simulink model "Pedal_Interpretation_exe"  (Simulink 7.0)
settings: Solver=ode4  StartTime=0.0  StopTime=88  FixedStep=0.01  RelTol=1e-3
InitFcn:
  | PedalInterp_para
values from neighbouring files (symbols this model uses):
  ped_min = 5    [PedalInterp_para.m]
  T_max_Brake = 4000    [PedalInterp_para.m]
  TI = 0    [PAS_callback.m]
undefined symbols (not defined in the file or in its folder): fzgbib, m_ab_100pro, m_ab_70pro, PedalInterpretation, v_bereich
libraries: simulink x320
(part 8 of 23)

== system Pedal_Interpretation_exe/Validation Functions/SR-PI-02.2 Acceleration pedal interpretation/v = const & phi_Acc increases & T_des_Drive < 0/PS ==
  A TI1 : Inport  OutDataType=sfix(16)  OutScaling=2^0
  A TI2 : Inport  Port=2  OutDataType=sfix(16)  OutScaling=2^0
  A TI3 : Inport  Port=3  OutDataType=sfix(16)  OutScaling=2^0
  AND : Logic  Inputs=4  AllPortsSameDT=off  OutDataTypeMode=boolean
  Bus Creator : BusCreator  Inputs=3
  Data Type Conversion : DataTypeConversion  OutDataType=sfix(16)  OutScaling=2^0
  Data Type Conversion1 : DataTypeConversion  OutDataType=sfix(16)  OutScaling=2^0
  Data Type Conversion2 : DataTypeConversion  OutDataType=sfix(16)  OutScaling=2^0
  Max Delay A : Subsystem  TreatAsAtomicUnit=on  mask{Delay=2}
      mask prompts: Delay "Delay (in simulation steps) for the input signal:"
      mask init:
      | %set_param([gcb '/Discrete Transfer Fcn'],'Denominator',['[' num2str([1 zeros(1,str2double(get_param(gcb,'Delay')))]) ']']);
      mask CallbackString:
      | Delay = str2double(get_param(gcb,'Delay'));
      | if Delay < 0
      |     set_param(gcb,'Delay','0');
      |     error('Only non-negative delays are possible (causality).');
      |     set_param([gcb '/Delay'],'Value','0');
      | elseif Delay == 0
      |     set_param([gcb '/Delay'],'Value','0');
      | else
      |     set_param([gcb '/Integer Delay'],'NumDelays',num2str(Delay));
      |     set_param([gcb '/Delay'],'Value',num2str(Delay));
      | end
      mask Display: text(0.5,0.5,['z^{ ' num2str((-1)*str2double(get_param(gcb,'Delay'))) '}'],'texmode','on');
  Max Delay R : Subsystem  TreatAsAtomicUnit=on  mask{Delay=2}
      mask prompts: Delay "Delay (in simulation steps) for the input signal:"
      mask init:
      | %set_param([gcb '/Discrete Transfer Fcn'],'Denominator',['[' num2str([1 zeros(1,str2double(get_param(gcb,'Delay')))]) ']']);
      mask CallbackString:
      | Delay = str2double(get_param(gcb,'Delay'));
      | if Delay < 0
      |     set_param(gcb,'Delay','0');
      |     error('Only non-negative delays are possible (causality).');
      |     set_param([gcb '/Delay'],'Value','0');
      | elseif Delay == 0
      |     set_param([gcb '/Delay'],'Value','0');
      | else
      |     set_param([gcb '/Integer Delay'],'NumDelays',num2str(Delay));
      |     set_param([gcb '/Delay'],'Value',num2str(Delay));
      | end
      mask Display: text(0.5,0.5,['z^{ ' num2str((-1)*str2double(get_param(gcb,'Delay'))) '}'],'texmode','on');
  Max Delay T : Subsystem  TreatAsAtomicUnit=on  mask{Delay=2}
      mask prompts: Delay "Delay (in simulation steps) for the input signal:"
      mask init:
      | %set_param([gcb '/Discrete Transfer Fcn'],'Denominator',['[' num2str([1 zeros(1,str2double(get_param(gcb,'Delay')))]) ']']);
      mask CallbackString:
      | Delay = str2double(get_param(gcb,'Delay'));
      | if Delay < 0
      |     set_param(gcb,'Delay','0');
      |     error('Only non-negative delays are possible (causality).');
      |     set_param([gcb '/Delay'],'Value','0');
      | elseif Delay == 0
      |     set_param([gcb '/Delay'],'Value','0');
      | else
      |     set_param([gcb '/Integer Delay'],'NumDelays',num2str(Delay));
      |     set_param([gcb '/Delay'],'Value',num2str(Delay));
      | end
      mask Display: text(0.5,0.5,['z^{ ' num2str((-1)*str2double(get_param(gcb,'Delay'))) '}'],'texmode','on');
  OR - AND : Subsystem
  TDD : Subsystem
  TI : Subsystem
  TID : Subsystem
  Precond : Outport  OutDataType=sfix(16)  OutScaling=2^0
  wires:
  TDD/2(T) -> AND/4
  TID/2(T) -> Max Delay T/1(In1)
  TID/1(A) -> Max Delay A/1(In1)
  Bus Creator/1 -> Precond/1
  Data Type Conversion/1 -> Bus Creator/1  "A"
  Data Type Conversion1/1 -> Bus Creator/2  "T"
  TDD/1(A) -> AND/3
  Max Delay T/1(Out1) -> Data Type Conversion1/1
  Max Delay R/1(Out1) -> AND/1
  Max Delay A/1(Out1) -> Data Type Conversion/1
  AND/1 -> Data Type Conversion2/1
  OR - AND/2(AND) -> TID/2(R AND), Max Delay R/1(In1)
  OR - AND/1(OR) -> TID/1(R OR)
  TI/1(A) -> AND/2
  Data Type Conversion2/1 -> Bus Creator/3  "R"
  A TI1/1 -> TI/1(A1)
  A TI2/1 -> TI/2(A2)
  A TI3/1 -> TI/3(A3)

== system Pedal_Interpretation_exe/Validation Functions/SR-PI-02.2 Acceleration pedal interpretation/v = const & phi_Acc increases & T_des_Drive < 0/Range - Gap Relative tolerance Precond ==
  Signal : Inport  OutDataType=sfix(16)  OutScaling=2^0
  Reference : Inport  Port=2  OutDataType=sfix(16)  OutScaling=2^0
  Abs : Abs
  Abs1 : Abs
  Add : Sum  Inputs=+-  OutDataType=sfix(16)  OutScaling=2^-10
  Divide1 : Product  Inputs=**/  OutDataType=sfix(16)  OutScaling=2^-10
  Max : Constant  Value=100  OutDataType=sfix(16)  OutScaling=2^0
  Relational Operator : RelationalOperator  Operator=<=  LogicOutDataTypeMode=boolean
  Relative Tolerance : Constant  OutDataType=sfix(16)  OutScaling=2^0
  Activate : Outport  OutDataType=sfix(16)  OutScaling=2^0
  wires:
  Abs/1 -> Relational Operator/1
  Add/1 -> Abs/1
  Signal/1 -> Add/1
  Reference/1 -> Add/2, Abs1/1
  Divide1/1 -> Relational Operator/2
  Max/1 -> Divide1/3
  Relative Tolerance/1 -> Divide1/2
  Relational Operator/1 -> Activate/1
  Abs1/1 -> Divide1/1

== system Pedal_Interpretation_exe/Validation Functions/SR-PI-02.2 Acceleration pedal interpretation/v = const & phi_Acc increases & T_des_Drive < 0/Range - Gap Relative tolerance Precond1 ==
  Signal : Inport  OutDataType=sfix(16)  OutScaling=2^0
  Reference : Inport  Port=2  OutDataType=sfix(16)  OutScaling=2^0
  Abs : Abs
  Abs1 : Abs
  Add : Sum  Inputs=+-  OutDataType=sfix(16)  OutScaling=2^-10
  Divide1 : Product  Inputs=**/  OutDataType=sfix(16)  OutScaling=2^-10
  Max : Constant  Value=100  OutDataType=sfix(16)  OutScaling=2^0
  Relational Operator : RelationalOperator  Operator=<=  LogicOutDataTypeMode=boolean
  Relative Tolerance : Constant  OutDataType=sfix(16)  OutScaling=2^0
  Activate : Outport  OutDataType=sfix(16)  OutScaling=2^0
  wires:
  Abs/1 -> Relational Operator/1
  Add/1 -> Abs/1
  Signal/1 -> Add/1
  Reference/1 -> Add/2, Abs1/1
  Divide1/1 -> Relational Operator/2
  Max/1 -> Divide1/3
  Relative Tolerance/1 -> Divide1/2
  Relational Operator/1 -> Activate/1
  Abs1/1 -> Divide1/1

== system Pedal_Interpretation_exe/Validation Functions/SR-PI-02.2 Acceleration pedal interpretation/v = const & phi_Acc increases & T_des_Drive >= 0/Bound Precond ==
  Signal : Inport  OutDataType=sfix(16)  OutScaling=2^0
  Reference : Inport  Port=2  OutDataType=sfix(16)  OutScaling=2^0
  RelOp : RelationalOperator  LogicOutDataTypeMode=Specify via dialog
  Activate : Outport  OutDataType=sfix(16)  OutScaling=2^0
  wires:
  Reference/1 -> RelOp/2
  RelOp/1 -> Activate/1
  Signal/1 -> RelOp/1

== system Pedal_Interpretation_exe/Validation Functions/SR-PI-02.2 Acceleration pedal interpretation/v = const & phi_Acc increases & T_des_Drive >= 0/Detect constant ==
  Signal : Inport  OutDataType=sfix(16)  OutScaling=2^0
  Clock : Clock
      settings: Decimation=10
  Constant1 : Constant  Value=0  OutDataTypeMode=boolean  OutDataType=sfix(16)  OutScaling=2^0
  Memory : Memory
  Relative tolerance : Subsystem
  Switch : Switch  Criteria=u2 > Threshold
  Constant : Outport  OutDataType=sfix(16)  OutScaling=2^0
  wires:
  Signal/1 -> Memory/1, Relative tolerance/1(sig)
  Memory/1 -> Relative tolerance/2(ref)
  Constant1/1 -> Switch/3
  Clock/1 -> Switch/2
  Relative tolerance/1(sig == ref) -> Switch/1
  Switch/1 -> Constant/1

== system Pedal_Interpretation_exe/Validation Functions/SR-PI-02.2 Acceleration pedal interpretation/v = const & phi_Acc increases & T_des_Drive >= 0/Detect increase ==
  Signal : Inport  OutDataType=sfix(16)  OutScaling=2^0
  Clock : Clock
      settings: Decimation=10
  Memory : Memory
  Relational Operator : RelationalOperator  Operator=>  LogicOutDataTypeMode=Specify via dialog
  Switch : Switch  Criteria=u2 > Threshold
  Increase : Outport  OutDataType=sfix(16)  OutScaling=2^0
  wires:
  Signal/1 -> Relational Operator/1, Memory/1, Switch/3
  Relational Operator/1 -> Increase/1
  Clock/1 -> Switch/2
  Memory/1 -> Switch/1
  Switch/1 -> Relational Operator/2

== system Pedal_Interpretation_exe/Validation Functions/SR-PI-02.2 Acceleration pedal interpretation/v = const & phi_Acc increases & T_des_Drive >= 0/PS ==
  A TI1 : Inport  OutDataType=sfix(16)  OutScaling=2^0
  A TI2 : Inport  Port=2  OutDataType=sfix(16)  OutScaling=2^0
  A TI3 : Inport  Port=3  OutDataType=sfix(16)  OutScaling=2^0
  AND : Logic  Inputs=4  AllPortsSameDT=off  OutDataTypeMode=boolean
  Bus Creator : BusCreator  Inputs=3
  Data Type Conversion : DataTypeConversion  OutDataType=sfix(16)  OutScaling=2^0
  Data Type Conversion1 : DataTypeConversion  OutDataType=sfix(16)  OutScaling=2^0
  Data Type Conversion2 : DataTypeConversion  OutDataType=sfix(16)  OutScaling=2^0
  Max Delay A : Subsystem  TreatAsAtomicUnit=on  mask{Delay=2}
      mask prompts: Delay "Delay (in simulation steps) for the input signal:"
      mask init:
      | %set_param([gcb '/Discrete Transfer Fcn'],'Denominator',['[' num2str([1 zeros(1,str2double(get_param(gcb,'Delay')))]) ']']);
      mask CallbackString:
      | Delay = str2double(get_param(gcb,'Delay'));
      | if Delay < 0
      |     set_param(gcb,'Delay','0');
      |     error('Only non-negative delays are possible (causality).');
      |     set_param([gcb '/Delay'],'Value','0');
      | elseif Delay == 0
      |     set_param([gcb '/Delay'],'Value','0');
      | else
      |     set_param([gcb '/Integer Delay'],'NumDelays',num2str(Delay));
      |     set_param([gcb '/Delay'],'Value',num2str(Delay));
      | end
      mask Display: text(0.5,0.5,['z^{ ' num2str((-1)*str2double(get_param(gcb,'Delay'))) '}'],'texmode','on');
  Max Delay R : Subsystem  TreatAsAtomicUnit=on  mask{Delay=2}
      mask prompts: Delay "Delay (in simulation steps) for the input signal:"
      mask init:
      | %set_param([gcb '/Discrete Transfer Fcn'],'Denominator',['[' num2str([1 zeros(1,str2double(get_param(gcb,'Delay')))]) ']']);
      mask CallbackString:
      | Delay = str2double(get_param(gcb,'Delay'));
      | if Delay < 0
      |     set_param(gcb,'Delay','0');
      |     error('Only non-negative delays are possible (causality).');
      |     set_param([gcb '/Delay'],'Value','0');
      | elseif Delay == 0
      |     set_param([gcb '/Delay'],'Value','0');
      | else
      |     set_param([gcb '/Integer Delay'],'NumDelays',num2str(Delay));
      |     set_param([gcb '/Delay'],'Value',num2str(Delay));
      | end
      mask Display: text(0.5,0.5,['z^{ ' num2str((-1)*str2double(get_param(gcb,'Delay'))) '}'],'texmode','on');
  Max Delay T : Subsystem  TreatAsAtomicUnit=on  mask{Delay=2}
      mask prompts: Delay "Delay (in simulation steps) for the input signal:"
      mask init:
      | %set_param([gcb '/Discrete Transfer Fcn'],'Denominator',['[' num2str([1 zeros(1,str2double(get_param(gcb,'Delay')))]) ']']);
      mask CallbackString:
      | Delay = str2double(get_param(gcb,'Delay'));
      | if Delay < 0
      |     set_param(gcb,'Delay','0');
      |     error('Only non-negative delays are possible (causality).');
      |     set_param([gcb '/Delay'],'Value','0');
      | elseif Delay == 0
      |     set_param([gcb '/Delay'],'Value','0');
      | else
      |     set_param([gcb '/Integer Delay'],'NumDelays',num2str(Delay));
      |     set_param([gcb '/Delay'],'Value',num2str(Delay));
      | end
      mask Display: text(0.5,0.5,['z^{ ' num2str((-1)*str2double(get_param(gcb,'Delay'))) '}'],'texmode','on');
  OR - AND : Subsystem
  TDD : Subsystem
  TI : Subsystem
  TID : Subsystem
  Precond : Outport  OutDataType=sfix(16)  OutScaling=2^0
  wires:
  TDD/2(T) -> AND/4
  TID/2(T) -> Max Delay T/1(In1)
  TID/1(A) -> Max Delay A/1(In1)
  Bus Creator/1 -> Precond/1
  Data Type Conversion/1 -> Bus Creator/1  "A"
  Data Type Conversion1/1 -> Bus Creator/2  "T"
  TDD/1(A) -> AND/3
  Max Delay T/1(Out1) -> Data Type Conversion1/1
  Max Delay R/1(Out1) -> AND/1
  Max Delay A/1(Out1) -> Data Type Conversion/1
  AND/1 -> Data Type Conversion2/1
  OR - AND/2(AND) -> TID/2(R AND), Max Delay R/1(In1)
  OR - AND/1(OR) -> TID/1(R OR)
  TI/1(A) -> AND/2
  Data Type Conversion2/1 -> Bus Creator/3  "R"
  A TI1/1 -> TI/1(A1)
  A TI2/1 -> TI/2(A2)
  A TI3/1 -> TI/3(A3)

== system Pedal_Interpretation_exe/Validation Functions/SR-PI-02.2 Acceleration pedal interpretation/v = const & phi_Acc increases & T_des_Drive >= 0/Range - Gap Relative tolerance Precond ==
  Signal : Inport  OutDataType=sfix(16)  OutScaling=2^0
  Reference : Inport  Port=2  OutDataType=sfix(16)  OutScaling=2^0
  Abs : Abs
  Abs1 : Abs
  Add : Sum  Inputs=+-  OutDataType=sfix(16)  OutScaling=2^-10
  Divide1 : Product  Inputs=**/  OutDataType=sfix(16)  OutScaling=2^-10
  Max : Constant  Value=100  OutDataType=sfix(16)  OutScaling=2^0
  Relational Operator : RelationalOperator  Operator=<=  LogicOutDataTypeMode=boolean
  Relative Tolerance : Constant  OutDataType=sfix(16)  OutScaling=2^0
  Activate : Outport  OutDataType=sfix(16)  OutScaling=2^0
  wires:
  Abs/1 -> Relational Operator/1
  Add/1 -> Abs/1
  Signal/1 -> Add/1
  Reference/1 -> Add/2, Abs1/1
  Divide1/1 -> Relational Operator/2
  Max/1 -> Divide1/3
  Relative Tolerance/1 -> Divide1/2
  Relational Operator/1 -> Activate/1
  Abs1/1 -> Divide1/1

== system Pedal_Interpretation_exe/Validation Functions/SR-PI-02.2 Acceleration pedal interpretation/v = const & phi_Acc increases & T_des_Drive >= 0/Range - Gap Relative tolerance Precond1 ==
  Signal : Inport  OutDataType=sfix(16)  OutScaling=2^0
  Reference : Inport  Port=2  OutDataType=sfix(16)  OutScaling=2^0
  Abs : Abs
  Abs1 : Abs
  Add : Sum  Inputs=+-  OutDataType=sfix(16)  OutScaling=2^-10
  Divide1 : Product  Inputs=**/  OutDataType=sfix(16)  OutScaling=2^-10
  Max : Constant  Value=100  OutDataType=sfix(16)  OutScaling=2^0
  Relational Operator : RelationalOperator  Operator=<=  LogicOutDataTypeMode=boolean
  Relative Tolerance : Constant  OutDataType=sfix(16)  OutScaling=2^0
  Activate : Outport  OutDataType=sfix(16)  OutScaling=2^0
  wires:
  Abs/1 -> Relational Operator/1
  Add/1 -> Abs/1
  Signal/1 -> Add/1
  Reference/1 -> Add/2, Abs1/1
  Divide1/1 -> Relational Operator/2
  Max/1 -> Divide1/3
  Relative Tolerance/1 -> Divide1/2
  Relational Operator/1 -> Activate/1
  Abs1/1 -> Divide1/1

== system Pedal_Interpretation_exe/Validation Functions/SR-PI-02.2 Acceleration pedal interpretation/v increases & phi_Acc = const & T_des_Drive >= 0/Bound Precond ==
  Signal : Inport  OutDataType=sfix(16)  OutScaling=2^0
  Reference : Inport  Port=2  OutDataType=sfix(16)  OutScaling=2^0
  RelOp : RelationalOperator  LogicOutDataTypeMode=Specify via dialog
  Activate : Outport  OutDataType=sfix(16)  OutScaling=2^0
  wires:
  Reference/1 -> RelOp/2
  RelOp/1 -> Activate/1
  Signal/1 -> RelOp/1

== system Pedal_Interpretation_exe/Validation Functions/SR-PI-02.2 Acceleration pedal interpretation/v increases & phi_Acc = const & T_des_Drive >= 0/Detect constant ==
  Signal : Inport  OutDataType=sfix(16)  OutScaling=2^0
  Clock : Clock
      settings: Decimation=10
  Constant1 : Constant  Value=0  OutDataTypeMode=boolean  OutDataType=sfix(16)  OutScaling=2^0
  Memory : Memory
  Relative tolerance : Subsystem
  Switch : Switch  Criteria=u2 > Threshold
  Constant : Outport  OutDataType=sfix(16)  OutScaling=2^0
  wires:
  Signal/1 -> Memory/1, Relative tolerance/1(sig)
  Memory/1 -> Relative tolerance/2(ref)
  Constant1/1 -> Switch/3
  Clock/1 -> Switch/2
  Relative tolerance/1(sig == ref) -> Switch/1
  Switch/1 -> Constant/1

== system Pedal_Interpretation_exe/Validation Functions/SR-PI-02.2 Acceleration pedal interpretation/v increases & phi_Acc = const & T_des_Drive >= 0/Detect increase ==
  Signal : Inport  OutDataType=sfix(16)  OutScaling=2^0
  Clock : Clock
      settings: Decimation=10
  Memory : Memory
  Relational Operator : RelationalOperator  Operator=>  LogicOutDataTypeMode=Specify via dialog
  Switch : Switch  Criteria=u2 > Threshold
  Increase : Outport  OutDataType=sfix(16)  OutScaling=2^0
  wires:
  Signal/1 -> Relational Operator/1, Memory/1, Switch/3
  Relational Operator/1 -> Increase/1
  Clock/1 -> Switch/2
  Memory/1 -> Switch/1
  Switch/1 -> Relational Operator/2

== system Pedal_Interpretation_exe/Validation Functions/SR-PI-02.2 Acceleration pedal interpretation/v increases & phi_Acc = const & T_des_Drive >= 0/PS ==
  A TI1 : Inport  OutDataType=sfix(16)  OutScaling=2^0
  A TI2 : Inport  Port=2  OutDataType=sfix(16)  OutScaling=2^0
  A TI3 : Inport  Port=3  OutDataType=sfix(16)  OutScaling=2^0
  AND : Logic  Inputs=4  AllPortsSameDT=off  OutDataTypeMode=boolean
  Bus Creator : BusCreator  Inputs=3
  Data Type Conversion : DataTypeConversion  OutDataType=sfix(16)  OutScaling=2^0
  Data Type Conversion1 : DataTypeConversion  OutDataType=sfix(16)  OutScaling=2^0
  Data Type Conversion2 : DataTypeConversion  OutDataType=sfix(16)  OutScaling=2^0
  Max Delay A : Subsystem  TreatAsAtomicUnit=on  mask{Delay=2}
      mask prompts: Delay "Delay (in simulation steps) for the input signal:"
      mask init:
      | %set_param([gcb '/Discrete Transfer Fcn'],'Denominator',['[' num2str([1 zeros(1,str2double(get_param(gcb,'Delay')))]) ']']);
      mask CallbackString:
      | Delay = str2double(get_param(gcb,'Delay'));
      | if Delay < 0
      |     set_param(gcb,'Delay','0');
      |     error('Only non-negative delays are possible (causality).');
      |     set_param([gcb '/Delay'],'Value','0');
      | elseif Delay == 0
      |     set_param([gcb '/Delay'],'Value','0');
      | else
      |     set_param([gcb '/Integer Delay'],'NumDelays',num2str(Delay));
      |     set_param([gcb '/Delay'],'Value',num2str(Delay));
      | end
      mask Display: text(0.5,0.5,['z^{ ' num2str((-1)*str2double(get_param(gcb,'Delay'))) '}'],'texmode','on');
  Max Delay R : Subsystem  TreatAsAtomicUnit=on  mask{Delay=2}
      mask prompts: Delay "Delay (in simulation steps) for the input signal:"
      mask init:
      | %set_param([gcb '/Discrete Transfer Fcn'],'Denominator',['[' num2str([1 zeros(1,str2double(get_param(gcb,'Delay')))]) ']']);
      mask CallbackString:
      | Delay = str2double(get_param(gcb,'Delay'));
      | if Delay < 0
      |     set_param(gcb,'Delay','0');
      |     error('Only non-negative delays are possible (causality).');
      |     set_param([gcb '/Delay'],'Value','0');
      | elseif Delay == 0
      |     set_param([gcb '/Delay'],'Value','0');
      | else
      |     set_param([gcb '/Integer Delay'],'NumDelays',num2str(Delay));
      |     set_param([gcb '/Delay'],'Value',num2str(Delay));
      | end
      mask Display: text(0.5,0.5,['z^{ ' num2str((-1)*str2double(get_param(gcb,'Delay'))) '}'],'texmode','on');
  Max Delay T : Subsystem  TreatAsAtomicUnit=on  mask{Delay=2}
      mask prompts: Delay "Delay (in simulation steps) for the input signal:"
      mask init:
      | %set_param([gcb '/Discrete Transfer Fcn'],'Denominator',['[' num2str([1 zeros(1,str2double(get_param(gcb,'Delay')))]) ']']);
      mask CallbackString:
      | Delay = str2double(get_param(gcb,'Delay'));
      | if Delay < 0
      |     set_param(gcb,'Delay','0');
      |     error('Only non-negative delays are possible (causality).');
      |     set_param([gcb '/Delay'],'Value','0');
      | elseif Delay == 0
      |     set_param([gcb '/Delay'],'Value','0');
      | else
      |     set_param([gcb '/Integer Delay'],'NumDelays',num2str(Delay));
      |     set_param([gcb '/Delay'],'Value',num2str(Delay));
      | end
      mask Display: text(0.5,0.5,['z^{ ' num2str((-1)*str2double(get_param(gcb,'Delay'))) '}'],'texmode','on');
  OR - AND : Subsystem
  TDD : Subsystem
  TI : Subsystem
  TID : Subsystem
  Precond : Outport  OutDataType=sfix(16)  OutScaling=2^0
  wires:
  TDD/2(T) -> AND/4
  TID/2(T) -> Max Delay T/1(In1)
  TID/1(A) -> Max Delay A/1(In1)
  Bus Creator/1 -> Precond/1
  Data Type Conversion/1 -> Bus Creator/1  "A"
  Data Type Conversion1/1 -> Bus Creator/2  "T"
  TDD/1(A) -> AND/3
  Max Delay T/1(Out1) -> Data Type Conversion1/1
  Max Delay R/1(Out1) -> AND/1
  Max Delay A/1(Out1) -> Data Type Conversion/1
  AND/1 -> Data Type Conversion2/1
  OR - AND/2(AND) -> TID/2(R AND), Max Delay R/1(In1)
  OR - AND/1(OR) -> TID/1(R OR)
  TI/1(A) -> AND/2
  Data Type Conversion2/1 -> Bus Creator/3  "R"
  A TI1/1 -> TI/1(A1)
  A TI2/1 -> TI/2(A2)
  A TI3/1 -> TI/3(A3)

== system Pedal_Interpretation_exe/Validation Functions/SR-PI-02.2 Acceleration pedal interpretation/v increases & phi_Acc = const & T_des_Drive >= 0/Range - Gap Relative tolerance Precond ==
  Signal : Inport  OutDataType=sfix(16)  OutScaling=2^0
  Reference : Inport  Port=2  OutDataType=sfix(16)  OutScaling=2^0
  Abs : Abs
  Abs1 : Abs
  Add : Sum  Inputs=+-  OutDataType=sfix(16)  OutScaling=2^-10
  Divide1 : Product  Inputs=**/  OutDataType=sfix(16)  OutScaling=2^-10
  Max : Constant  Value=100  OutDataType=sfix(16)  OutScaling=2^0
  Relational Operator : RelationalOperator  Operator=<=  LogicOutDataTypeMode=boolean
  Relative Tolerance : Constant  OutDataType=sfix(16)  OutScaling=2^0
  Activate : Outport  OutDataType=sfix(16)  OutScaling=2^0
  wires:
  Abs/1 -> Relational Operator/1
  Add/1 -> Abs/1
  Signal/1 -> Add/1
  Reference/1 -> Add/2, Abs1/1
  Divide1/1 -> Relational Operator/2
  Max/1 -> Divide1/3
  Relative Tolerance/1 -> Divide1/2
  Relational Operator/1 -> Activate/1
  Abs1/1 -> Divide1/1

== system Pedal_Interpretation_exe/Validation Functions/SR-PI-02.2 Acceleration pedal interpretation/v increases & phi_Acc = const & T_des_Drive >= 0/Range - Gap Relative tolerance Precond1 ==
  Signal : Inport  OutDataType=sfix(16)  OutScaling=2^0
  Reference : Inport  Port=2  OutDataType=sfix(16)  OutScaling=2^0
  Abs : Abs
  Abs1 : Abs
  Add : Sum  Inputs=+-  OutDataType=sfix(16)  OutScaling=2^-10
  Divide1 : Product  Inputs=**/  OutDataType=sfix(16)  OutScaling=2^-10
  Max : Constant  Value=100  OutDataType=sfix(16)  OutScaling=2^0
  Relational Operator : RelationalOperator  Operator=<=  LogicOutDataTypeMode=boolean
  Relative Tolerance : Constant  OutDataType=sfix(16)  OutScaling=2^0
  Activate : Outport  OutDataType=sfix(16)  OutScaling=2^0
  wires:
  Abs/1 -> Relational Operator/1
  Add/1 -> Abs/1
  Signal/1 -> Add/1
  Reference/1 -> Add/2, Abs1/1
  Divide1/1 -> Relational Operator/2
  Max/1 -> Divide1/3
  Relative Tolerance/1 -> Divide1/2
  Relational Operator/1 -> Activate/1
  Abs1/1 -> Divide1/1

== system Pedal_Interpretation_exe/TestData 1/SR-PI-01.1 Brake Pedal recognition/phi_Brake < ped_min/Generate decrease 2/Generate  limited decrease for partition1 variant1 1 ==
  Repeating Sequence : Subsystem  mask(Repeating table){rep_seq_t=[0 T], rep_seq_y=[X0 XF]}
      mask prompts: rep_seq_t "Time values:"; rep_seq_y "Output values:"
      mask help: Output a repeating sequence of numbers specified in a table of time-value pairs. Values of time should be monotonically increasing.
      mask init:
      | if (length(rep_seq_t) ~= length(rep_seq_y)),
      |   error('Length of time vector and output vector must be the same.')
      | end
      | dbl_rep_seq_t = double(rep_seq_t);
      | dbl_rep_seq_y = double(rep_seq_y);
      | period = max(dbl_rep_seq_t) - min(dbl_rep_seq_t);
      | s = round(length(dbl_rep_seq_t)/50);
      | if s > 0
      |   pts = [1:s:length(dbl_rep_seq_t)];
      |   L   = length(pts);
      | else
      |   L   = length(dbl_rep_seq_t);
      |   pts = [1:L];
      | end
      | 
      | disp_seq_t = reshape(dbl_rep_seq_t(pts),L,1);
      | disp_seq_y = reshape(dbl_rep_seq_y(pts),L,1);
      | disp_period = max(disp_seq_t) - min(disp_seq_t);
      | 
      | disp_seq_t  = repmat(disp_seq_t,1,3) + (ones(L,1)*(disp_period*[0,1,2]));
      | disp_seq_t = [ disp_seq_t(:); disp_seq_t(end) ];
      | disp_seq_y = repmat(disp_seq_y,1,3);
      | disp_seq_y = [ disp_seq_y(:); disp_seq_y(1) ];
      mask Help: Repeats cycle given in table. Time values should be monotonically increasing.
      mask Display: plot( disp_seq_t, disp_seq_y )
  Out1 : Outport  OutDataType=sfix(16)  OutScaling=2^0
  wires:
  Repeating Sequence/1(Out1) -> Out1/1

== system Pedal_Interpretation_exe/TestData 1/SR-PI-01.1 Brake Pedal recognition/phi_Brake < ped_min/Generate decrease 2/Generate  limited decrease for partition1 variant2 1 ==
  Repeating Sequence : Subsystem  mask(Repeating table){rep_seq_t=[0 T], rep_seq_y=[X0 XF]}
      mask prompts: rep_seq_t "Time values:"; rep_seq_y "Output values:"
      mask help: Output a repeating sequence of numbers specified in a table of time-value pairs. Values of time should be monotonically increasing.
      mask init: same as Pedal_Interpretation_exe/TestData 1/SR-PI-01.1 Brake Pedal recognition/phi_Brake < ped_min/Generate decrease 2/Generate  limited decrease for partition1 variant1 1/Repeating Sequence
      mask Help: Repeats cycle given in table. Time values should be monotonically increasing.
      mask Display: plot( disp_seq_t, disp_seq_y )
  Out1 : Outport  OutDataType=sfix(16)  OutScaling=2^0
  wires:
  Repeating Sequence/1(Out1) -> Out1/1

== system Pedal_Interpretation_exe/TestData 1/SR-PI-01.1 Brake Pedal recognition/phi_Brake < ped_min/Generate decrease 2/TestDataVariants Sequence ==
  Constant : Constant  Value=2  OutDataType=sfix(16)  OutScaling=2^0
  Relational Operator : RelationalOperator  Operator=<=  LogicOutDataTypeMode=boolean
  Switch : Switch  Criteria=u2 ~= 0  OutDataType=sfix(16)  OutScaling=2^0
  Out1 : Outport  OutDataType=sfix(16)  OutScaling=2^0
  wires:
  [A] -> Relational Operator/1, Switch/1
  Constant/1 -> Relational Operator/2, Switch/3
  Relational Operator/1 -> Switch/2
  Switch/1 -> Out1/1

== system Pedal_Interpretation_exe/TestData 1/SR-PI-01.1 Brake Pedal recognition/phi_Brake >= ped_min/Generate increase 2/Generate  limited increase for partition1 variant1 1 ==
  Repeating Sequence : Subsystem  mask(Repeating table){rep_seq_t=[0 T], rep_seq_y=[X0 XF]}
      mask prompts: rep_seq_t "Time values:"; rep_seq_y "Output values:"
      mask help: Output a repeating sequence of numbers specified in a table of time-value pairs. Values of time should be monotonically increasing.
      mask init: same as Pedal_Interpretation_exe/TestData 1/SR-PI-01.1 Brake Pedal recognition/phi_Brake < ped_min/Generate decrease 2/Generate  limited decrease for partition1 variant1 1/Repeating Sequence
      mask Help: Repeats cycle given in table. Time values should be monotonically increasing.
      mask Display: plot( disp_seq_t, disp_seq_y )
  Out1 : Outport  OutDataType=sfix(16)  OutScaling=2^0
  wires:
  Repeating Sequence/1(Out1) -> Out1/1

== system Pedal_Interpretation_exe/TestData 1/SR-PI-01.1 Brake Pedal recognition/phi_Brake >= ped_min/Generate increase 2/Generate  limited increase for partition1 variant2 1 ==
  Repeating Sequence : Subsystem  mask(Repeating table){rep_seq_t=[0 T], rep_seq_y=[X0 XF]}
      mask prompts: rep_seq_t "Time values:"; rep_seq_y "Output values:"
      mask help: Output a repeating sequence of numbers specified in a table of time-value pairs. Values of time should be monotonically increasing.
      mask init: same as Pedal_Interpretation_exe/TestData 1/SR-PI-01.1 Brake Pedal recognition/phi_Brake < ped_min/Generate decrease 2/Generate  limited decrease for partition1 variant1 1/Repeating Sequence
      mask Help: Repeats cycle given in table. Time values should be monotonically increasing.
      mask Display: plot( disp_seq_t, disp_seq_y )
  Out1 : Outport  OutDataType=sfix(16)  OutScaling=2^0
  wires:
  Repeating Sequence/1(Out1) -> Out1/1

== system Pedal_Interpretation_exe/TestData 1/SR-PI-01.1 Brake Pedal recognition/phi_Brake >= ped_min/Generate increase 2/TestDataVariants Sequence ==
  Constant : Constant  Value=2  OutDataType=sfix(16)  OutScaling=2^0
  Relational Operator : RelationalOperator  Operator=<=  LogicOutDataTypeMode=boolean
  Switch : Switch  Criteria=u2 ~= 0  OutDataType=sfix(16)  OutScaling=2^0
  Out1 : Outport  OutDataType=sfix(16)  OutScaling=2^0
  wires:
  [A] -> Relational Operator/1, Switch/1
  Constant/1 -> Relational Operator/2, Switch/3
  Relational Operator/1 -> Switch/2
  Switch/1 -> Out1/1

== system Pedal_Interpretation_exe/TestData 1/SR-PI-01.3 Acceleration Pedal recognition/phi_Acc < ped_min/Generate decrease 2/Generate  limited decrease for partition1 variant1 1 ==
  Repeating Sequence : Subsystem  mask(Repeating table){rep_seq_t=[0 T], rep_seq_y=[X0 XF]}
      mask prompts: rep_seq_t "Time values:"; rep_seq_y "Output values:"
      mask help: Output a repeating sequence of numbers specified in a table of time-value pairs. Values of time should be monotonically increasing.
      mask init: same as Pedal_Interpretation_exe/TestData 1/SR-PI-01.1 Brake Pedal recognition/phi_Brake < ped_min/Generate decrease 2/Generate  limited decrease for partition1 variant1 1/Repeating Sequence
      mask Help: Repeats cycle given in table. Time values should be monotonically increasing.
      mask Display: plot( disp_seq_t, disp_seq_y )
  Out1 : Outport  OutDataType=sfix(16)  OutScaling=2^0
  wires:
  Repeating Sequence/1(Out1) -> Out1/1

== system Pedal_Interpretation_exe/TestData 1/SR-PI-01.3 Acceleration Pedal recognition/phi_Acc < ped_min/Generate decrease 2/Generate  limited decrease for partition1 variant2 1 ==
  Repeating Sequence : Subsystem  mask(Repeating table){rep_seq_t=[0 T], rep_seq_y=[X0 XF]}
      mask prompts: rep_seq_t "Time values:"; rep_seq_y "Output values:"
      mask help: Output a repeating sequence of numbers specified in a table of time-value pairs. Values of time should be monotonically increasing.
      mask init: same as Pedal_Interpretation_exe/TestData 1/SR-PI-01.1 Brake Pedal recognition/phi_Brake < ped_min/Generate decrease 2/Generate  limited decrease for partition1 variant1 1/Repeating Sequence
      mask Help: Repeats cycle given in table. Time values should be monotonically increasing.
      mask Display: plot( disp_seq_t, disp_seq_y )
  Out1 : Outport  OutDataType=sfix(16)  OutScaling=2^0
  wires:
  Repeating Sequence/1(Out1) -> Out1/1

== system Pedal_Interpretation_exe/TestData 1/SR-PI-01.3 Acceleration Pedal recognition/phi_Acc < ped_min/Generate decrease 2/TestDataVariants Sequence ==
  Constant : Constant  Value=2  OutDataType=sfix(16)  OutScaling=2^0
  Relational Operator : RelationalOperator  Operator=<=  LogicOutDataTypeMode=boolean
  Switch : Switch  Criteria=u2 ~= 0  OutDataType=sfix(16)  OutScaling=2^0
  Out1 : Outport  OutDataType=sfix(16)  OutScaling=2^0
  wires:
  [A] -> Relational Operator/1, Switch/1
  Constant/1 -> Relational Operator/2, Switch/3
  Relational Operator/1 -> Switch/2
  Switch/1 -> Out1/1

== system Pedal_Interpretation_exe/TestData 1/SR-PI-01.3 Acceleration Pedal recognition/phi_Acc >= ped_min/Generate increase 2/Generate  limited increase for partition1 variant1 1 ==
  Repeating Sequence : Subsystem  mask(Repeating table){rep_seq_t=[0 T], rep_seq_y=[X0 XF]}
      mask prompts: rep_seq_t "Time values:"; rep_seq_y "Output values:"
      mask help: Output a repeating sequence of numbers specified in a table of time-value pairs. Values of time should be monotonically increasing.
      mask init: same as Pedal_Interpretation_exe/TestData 1/SR-PI-01.1 Brake Pedal recognition/phi_Brake < ped_min/Generate decrease 2/Generate  limited decrease for partition1 variant1 1/Repeating Sequence
      mask Help: Repeats cycle given in table. Time values should be monotonically increasing.
      mask Display: plot( disp_seq_t, disp_seq_y )
  Out1 : Outport  OutDataType=sfix(16)  OutScaling=2^0
  wires:
  Repeating Sequence/1(Out1) -> Out1/1

== system Pedal_Interpretation_exe/TestData 1/SR-PI-01.3 Acceleration Pedal recognition/phi_Acc >= ped_min/Generate increase 2/Generate  limited increase for partition1 variant2 1 ==
  Repeating Sequence : Subsystem  mask(Repeating table){rep_seq_t=[0 T], rep_seq_y=[X0 XF]}
      mask prompts: rep_seq_t "Time values:"; rep_seq_y "Output values:"
      mask help: Output a repeating sequence of numbers specified in a table of time-value pairs. Values of time should be monotonically increasing.
      mask init: same as Pedal_Interpretation_exe/TestData 1/SR-PI-01.1 Brake Pedal recognition/phi_Brake < ped_min/Generate decrease 2/Generate  limited decrease for partition1 variant1 1/Repeating Sequence
      mask Help: Repeats cycle given in table. Time values should be monotonically increasing.
      mask Display: plot( disp_seq_t, disp_seq_y )
  Out1 : Outport  OutDataType=sfix(16)  OutScaling=2^0
  wires:
  Repeating Sequence/1(Out1) -> Out1/1

== system Pedal_Interpretation_exe/TestData 1/SR-PI-01.3 Acceleration Pedal recognition/phi_Acc >= ped_min/Generate increase 2/TestDataVariants Sequence ==
  Constant : Constant  Value=2  OutDataType=sfix(16)  OutScaling=2^0
  Relational Operator : RelationalOperator  Operator=<=  LogicOutDataTypeMode=boolean
  Switch : Switch  Criteria=u2 ~= 0  OutDataType=sfix(16)  OutScaling=2^0
  Out1 : Outport  OutDataType=sfix(16)  OutScaling=2^0
  wires:
  [A] -> Relational Operator/1, Switch/1
  Constant/1 -> Relational Operator/2, Switch/3
  Relational Operator/1 -> Switch/2
  Switch/1 -> Out1/1

== system Pedal_Interpretation_exe/TestData 1/SR-PI-02.2 Acceleration pedal interpretation/v = const & phi_Acc = const/Generate constant 5/Generate  constant for partition1 variant1 1 ==
  Repeating Sequence : Subsystem  mask(Repeating table){rep_seq_t=[0 T], rep_seq_y=[X0 X0]}
      mask prompts: rep_seq_t "Time values:"; rep_seq_y "Output values:"
      mask help: Output a repeating sequence of numbers specified in a table of time-value pairs. Values of time should be monotonically increasing.
      mask init: same as Pedal_Interpretation_exe/TestData 1/SR-PI-01.1 Brake Pedal recognition/phi_Brake < ped_min/Generate decrease 2/Generate  limited decrease for partition1 variant1 1/Repeating Sequence
      mask Help: Repeats cycle given in table. Time values should be monotonically increasing.
      mask Display: plot( disp_seq_t, disp_seq_y )
  Out1 : Outport  OutDataType=sfix(16)  OutScaling=2^0
  wires:
  Repeating Sequence/1(Out1) -> Out1/1

== system Pedal_Interpretation_exe/TestData 1/SR-PI-02.2 Acceleration pedal interpretation/v = const & phi_Acc = const/Generate constant 5/Generate  constant for partition1 variant2 1 ==
  Repeating Sequence : Subsystem  mask(Repeating table){rep_seq_t=[0 T], rep_seq_y=[X0 X0]}
      mask prompts: rep_seq_t "Time values:"; rep_seq_y "Output values:"
      mask help: Output a repeating sequence of numbers specified in a table of time-value pairs. Values of time should be monotonically increasing.
      mask init: same as Pedal_Interpretation_exe/TestData 1/SR-PI-01.1 Brake Pedal recognition/phi_Brake < ped_min/Generate decrease 2/Generate  limited decrease for partition1 variant1 1/Repeating Sequence
      mask Help: Repeats cycle given in table. Time values should be monotonically increasing.
      mask Display: plot( disp_seq_t, disp_seq_y )
  Out1 : Outport  OutDataType=sfix(16)  OutScaling=2^0
  wires:
  Repeating Sequence/1(Out1) -> Out1/1

== system Pedal_Interpretation_exe/TestData 1/SR-PI-02.2 Acceleration pedal interpretation/v = const & phi_Acc = const/Generate constant 5/Generate  constant for partition1 variant3 1 ==
  Repeating Sequence : Subsystem  mask(Repeating table){rep_seq_t=[0 T], rep_seq_y=[X0 X0]}
      mask prompts: rep_seq_t "Time values:"; rep_seq_y "Output values:"
      mask help: Output a repeating sequence of numbers specified in a table of time-value pairs. Values of time should be monotonically increasing.
      mask init: same as Pedal_Interpretation_exe/TestData 1/SR-PI-01.1 Brake Pedal recognition/phi_Brake < ped_min/Generate decrease 2/Generate  limited decrease for partition1 variant1 1/Repeating Sequence
      mask Help: Repeats cycle given in table. Time values should be monotonically increasing.
      mask Display: plot( disp_seq_t, disp_seq_y )
  Out1 : Outport  OutDataType=sfix(16)  OutScaling=2^0
  wires:
  Repeating Sequence/1(Out1) -> Out1/1

== system Pedal_Interpretation_exe/TestData 1/SR-PI-02.2 Acceleration pedal interpretation/v = const & phi_Acc = const/Generate constant 5/Generate  constant for partition1 variant4 1 ==
  Repeating Sequence : Subsystem  mask(Repeating table){rep_seq_t=[0 T], rep_seq_y=[X0 X0]}
      mask prompts: rep_seq_t "Time values:"; rep_seq_y "Output values:"
      mask help: Output a repeating sequence of numbers specified in a table of time-value pairs. Values of time should be monotonically increasing.
      mask init: same as Pedal_Interpretation_exe/TestData 1/SR-PI-01.1 Brake Pedal recognition/phi_Brake < ped_min/Generate decrease 2/Generate  limited decrease for partition1 variant1 1/Repeating Sequence
      mask Help: Repeats cycle given in table. Time values should be monotonically increasing.
      mask Display: plot( disp_seq_t, disp_seq_y )
  Out1 : Outport  OutDataType=sfix(16)  OutScaling=2^0
  wires:
  Repeating Sequence/1(Out1) -> Out1/1

== system Pedal_Interpretation_exe/TestData 1/SR-PI-02.2 Acceleration pedal interpretation/v = const & phi_Acc = const/Generate constant 5/Generate  constant for partition1 variant5 1 ==
  Repeating Sequence : Subsystem  mask(Repeating table){rep_seq_t=[0 T], rep_seq_y=[X0 X0]}
      mask prompts: rep_seq_t "Time values:"; rep_seq_y "Output values:"
      mask help: Output a repeating sequence of numbers specified in a table of time-value pairs. Values of time should be monotonically increasing.
      mask init: same as Pedal_Interpretation_exe/TestData 1/SR-PI-01.1 Brake Pedal recognition/phi_Brake < ped_min/Generate decrease 2/Generate  limited decrease for partition1 variant1 1/Repeating Sequence
      mask Help: Repeats cycle given in table. Time values should be monotonically increasing.
      mask Display: plot( disp_seq_t, disp_seq_y )
  Out1 : Outport  OutDataType=sfix(16)  OutScaling=2^0
  wires:
  Repeating Sequence/1(Out1) -> Out1/1

== system Pedal_Interpretation_exe/TestData 1/SR-PI-02.2 Acceleration pedal interpretation/v = const & phi_Acc = const/Generate constant 5/TestDataVariants Sequence ==
  Constant : Constant  Value=5  OutDataType=sfix(16)  OutScaling=2^0
  Relational Operator : RelationalOperator  Operator=<=  LogicOutDataTypeMode=boolean
  Switch : Switch  Criteria=u2 ~= 0  OutDataType=sfix(16)  OutScaling=2^0
  Out1 : Outport  OutDataType=sfix(16)  OutScaling=2^0
  wires:
  [A] -> Relational Operator/1, Switch/1
  Constant/1 -> Relational Operator/2, Switch/3
  Relational Operator/1 -> Switch/2
  Switch/1 -> Out1/1

== system Pedal_Interpretation_exe/TestData 1/SR-PI-02.2 Acceleration pedal interpretation/v = const & phi_Acc = const/Generate constant 6/Generate  constant for partition1 variant1 1 ==
  Repeating Sequence : Subsystem  mask(Repeating table){rep_seq_t=[0 T], rep_seq_y=[X0 X0]}
      mask prompts: rep_seq_t "Time values:"; rep_seq_y "Output values:"
      mask help: Output a repeating sequence of numbers specified in a table of time-value pairs. Values of time should be monotonically increasing.
      mask init: same as Pedal_Interpretation_exe/TestData 1/SR-PI-01.1 Brake Pedal recognition/phi_Brake < ped_min/Generate decrease 2/Generate  limited decrease for partition1 variant1 1/Repeating Sequence
      mask Help: Repeats cycle given in table. Time values should be monotonically increasing.
      mask Display: plot( disp_seq_t, disp_seq_y )
  Out1 : Outport  OutDataType=sfix(16)  OutScaling=2^0
  wires:
  Repeating Sequence/1(Out1) -> Out1/1

== system Pedal_Interpretation_exe/TestData 1/SR-PI-02.2 Acceleration pedal interpretation/v = const & phi_Acc = const/Generate constant 6/Generate  constant for partition1 variant2 1 ==
  Repeating Sequence : Subsystem  mask(Repeating table){rep_seq_t=[0 T], rep_seq_y=[X0 X0]}
      mask prompts: rep_seq_t "Time values:"; rep_seq_y "Output values:"
      mask help: Output a repeating sequence of numbers specified in a table of time-value pairs. Values of time should be monotonically increasing.
      mask init: same as Pedal_Interpretation_exe/TestData 1/SR-PI-01.1 Brake Pedal recognition/phi_Brake < ped_min/Generate decrease 2/Generate  limited decrease for partition1 variant1 1/Repeating Sequence
      mask Help: Repeats cycle given in table. Time values should be monotonically increasing.
      mask Display: plot( disp_seq_t, disp_seq_y )
  Out1 : Outport  OutDataType=sfix(16)  OutScaling=2^0
  wires:
  Repeating Sequence/1(Out1) -> Out1/1

== system Pedal_Interpretation_exe/TestData 1/SR-PI-02.2 Acceleration pedal interpretation/v = const & phi_Acc = const/Generate constant 6/Generate  constant for partition1 variant3 1 ==
  Repeating Sequence : Subsystem  mask(Repeating table){rep_seq_t=[0 T], rep_seq_y=[X0 X0]}
      mask prompts: rep_seq_t "Time values:"; rep_seq_y "Output values:"
      mask help: Output a repeating sequence of numbers specified in a table of time-value pairs. Values of time should be monotonically increasing.
      mask init: same as Pedal_Interpretation_exe/TestData 1/SR-PI-01.1 Brake Pedal recognition/phi_Brake < ped_min/Generate decrease 2/Generate  limited decrease for partition1 variant1 1/Repeating Sequence
      mask Help: Repeats cycle given in table. Time values should be monotonically increasing.
      mask Display: plot( disp_seq_t, disp_seq_y )
  Out1 : Outport  OutDataType=sfix(16)  OutScaling=2^0
  wires:
  Repeating Sequence/1(Out1) -> Out1/1

== system Pedal_Interpretation_exe/TestData 1/SR-PI-02.2 Acceleration pedal interpretation/v = const & phi_Acc = const/Generate constant 6/TestDataVariants Sequence ==
  Constant : Constant  Value=3  OutDataType=sfix(16)  OutScaling=2^0
  Relational Operator : RelationalOperator  Operator=<=  LogicOutDataTypeMode=boolean
  Switch : Switch  Criteria=u2 ~= 0  OutDataType=sfix(16)  OutScaling=2^0
  Out1 : Outport  OutDataType=sfix(16)  OutScaling=2^0
  wires:
  [A] -> Relational Operator/1, Switch/1
  Constant/1 -> Relational Operator/2, Switch/3
  Relational Operator/1 -> Switch/2
  Switch/1 -> Out1/1

== system Pedal_Interpretation_exe/TestData 1/SR-PI-02.2 Acceleration pedal interpretation/v = const & phi_Acc decreases & T_des_Drive < 0/Generate constant 6/Generate  constant for partition1 variant1 1 ==
  Repeating Sequence : Subsystem  mask(Repeating table){rep_seq_t=[0 T], rep_seq_y=[X0 X0]}
      mask prompts: rep_seq_t "Time values:"; rep_seq_y "Output values:"
      mask help: Output a repeating sequence of numbers specified in a table of time-value pairs. Values of time should be monotonically increasing.
      mask init: same as Pedal_Interpretation_exe/TestData 1/SR-PI-01.1 Brake Pedal recognition/phi_Brake < ped_min/Generate decrease 2/Generate  limited decrease for partition1 variant1 1/Repeating Sequence
      mask Help: Repeats cycle given in table. Time values should be monotonically increasing.
      mask Display: plot( disp_seq_t, disp_seq_y )
  Out1 : Outport  OutDataType=sfix(16)  OutScaling=2^0
  wires:
  Repeating Sequence/1(Out1) -> Out1/1

== system Pedal_Interpretation_exe/TestData 1/SR-PI-02.2 Acceleration pedal interpretation/v = const & phi_Acc decreases & T_des_Drive < 0/Generate constant 6/Generate  constant for partition1 variant2 1 ==
  Repeating Sequence : Subsystem  mask(Repeating table){rep_seq_t=[0 T], rep_seq_y=[X0 X0]}
      mask prompts: rep_seq_t "Time values:"; rep_seq_y "Output values:"
      mask help: Output a repeating sequence of numbers specified in a table of time-value pairs. Values of time should be monotonically increasing.
      mask init: same as Pedal_Interpretation_exe/TestData 1/SR-PI-01.1 Brake Pedal recognition/phi_Brake < ped_min/Generate decrease 2/Generate  limited decrease for partition1 variant1 1/Repeating Sequence
      mask Help: Repeats cycle given in table. Time values should be monotonically increasing.
      mask Display: plot( disp_seq_t, disp_seq_y )
  Out1 : Outport  OutDataType=sfix(16)  OutScaling=2^0
  wires:
  Repeating Sequence/1(Out1) -> Out1/1

== system Pedal_Interpretation_exe/TestData 1/SR-PI-02.2 Acceleration pedal interpretation/v = const & phi_Acc decreases & T_des_Drive < 0/Generate constant 6/Generate  constant for partition1 variant3 1 ==
  Repeating Sequence : Subsystem  mask(Repeating table){rep_seq_t=[0 T], rep_seq_y=[X0 X0]}
      mask prompts: rep_seq_t "Time values:"; rep_seq_y "Output values:"
      mask help: Output a repeating sequence of numbers specified in a table of time-value pairs. Values of time should be monotonically increasing.
      mask init: same as Pedal_Interpretation_exe/TestData 1/SR-PI-01.1 Brake Pedal recognition/phi_Brake < ped_min/Generate decrease 2/Generate  limited decrease for partition1 variant1 1/Repeating Sequence
      mask Help: Repeats cycle given in table. Time values should be monotonically increasing.
      mask Display: plot( disp_seq_t, disp_seq_y )
  Out1 : Outport  OutDataType=sfix(16)  OutScaling=2^0
  wires:
  Repeating Sequence/1(Out1) -> Out1/1

== system Pedal_Interpretation_exe/TestData 1/SR-PI-02.2 Acceleration pedal interpretation/v = const & phi_Acc decreases & T_des_Drive < 0/Generate constant 6/Generate  constant for partition1 variant4 1 ==
  Repeating Sequence : Subsystem  mask(Repeating table){rep_seq_t=[0 T], rep_seq_y=[X0 X0]}
      mask prompts: rep_seq_t "Time values:"; rep_seq_y "Output values:"
      mask help: Output a repeating sequence of numbers specified in a table of time-value pairs. Values of time should be monotonically increasing.
      mask init: same as Pedal_Interpretation_exe/TestData 1/SR-PI-01.1 Brake Pedal recognition/phi_Brake < ped_min/Generate decrease 2/Generate  limited decrease for partition1 variant1 1/Repeating Sequence
      mask Help: Repeats cycle given in table. Time values should be monotonically increasing.
      mask Display: plot( disp_seq_t, disp_seq_y )
  Out1 : Outport  OutDataType=sfix(16)  OutScaling=2^0
  wires:
  Repeating Sequence/1(Out1) -> Out1/1

== system Pedal_Interpretation_exe/TestData 1/SR-PI-02.2 Acceleration pedal interpretation/v = const & phi_Acc decreases & T_des_Drive < 0/Generate constant 6/Generate  constant for partition1 variant5 1 ==
  Repeating Sequence : Subsystem  mask(Repeating table){rep_seq_t=[0 T], rep_seq_y=[X0 X0]}
      mask prompts: rep_seq_t "Time values:"; rep_seq_y "Output values:"
      mask help: Output a repeating sequence of numbers specified in a table of time-value pairs. Values of time should be monotonically increasing.
      mask init: same as Pedal_Interpretation_exe/TestData 1/SR-PI-01.1 Brake Pedal recognition/phi_Brake < ped_min/Generate decrease 2/Generate  limited decrease for partition1 variant1 1/Repeating Sequence
      mask Help: Repeats cycle given in table. Time values should be monotonically increasing.
      mask Display: plot( disp_seq_t, disp_seq_y )
  Out1 : Outport  OutDataType=sfix(16)  OutScaling=2^0
  wires:
  Repeating Sequence/1(Out1) -> Out1/1

== system Pedal_Interpretation_exe/TestData 1/SR-PI-02.2 Acceleration pedal interpretation/v = const & phi_Acc decreases & T_des_Drive < 0/Generate constant 6/TestDataVariants Sequence ==
  Constant : Constant  Value=5  OutDataType=sfix(16)  OutScaling=2^0
  Relational Operator : RelationalOperator  Operator=<=  LogicOutDataTypeMode=boolean
  Switch : Switch  Criteria=u2 ~= 0  OutDataType=sfix(16)  OutScaling=2^0
  Out1 : Outport  OutDataType=sfix(16)  OutScaling=2^0
  wires:
  [A] -> Relational Operator/1, Switch/1
  Constant/1 -> Relational Operator/2, Switch/3
  Relational Operator/1 -> Switch/2
  Switch/1 -> Out1/1

== system Pedal_Interpretation_exe/TestData 1/SR-PI-02.2 Acceleration pedal interpretation/v = const & phi_Acc decreases & T_des_Drive < 0/Generate decrease 7/Generate  limited decrease for partition1 variant1 1 ==
  Repeating Sequence : Subsystem  mask(Repeating table){rep_seq_t=[0 T], rep_seq_y=[X0 XF]}
      mask prompts: rep_seq_t "Time values:"; rep_seq_y "Output values:"
      mask help: Output a repeating sequence of numbers specified in a table of time-value pairs. Values of time should be monotonically increasing.
      mask init: same as Pedal_Interpretation_exe/TestData 1/SR-PI-01.1 Brake Pedal recognition/phi_Brake < ped_min/Generate decrease 2/Generate  limited decrease for partition1 variant1 1/Repeating Sequence
      mask Help: Repeats cycle given in table. Time values should be monotonically increasing.
      mask Display: plot( disp_seq_t, disp_seq_y )
  Out1 : Outport  OutDataType=sfix(16)  OutScaling=2^0
  wires:
  Repeating Sequence/1(Out1) -> Out1/1
